simulink model "FuelSecondary_harness"  (Simulink 7.7)
settings: Solver=FixedStepDiscrete  SolverMode=SingleTasking  StartTime=0.0  StopTime=100  FixedStep=srate  RelTol=1e-3
InitFcn:
  | if signalbuilder('FuelSecondary_harness/Signal_Builder','activegroup') == 1
  |   CD_FUEL_SECONDARY_FUNCTION.DataType = 'uint8';
  |   CD_FUEL_SECONDARY_FUNCTION.Value = 255;
  |   CD_FUEL_SECONDARY_FEEDBACK_FUNCTION.DataType = 'uint8';
  |   CD_FUEL_SECONDARY_FEEDBACK_FUNCTION.Value = 255;
  | elseif signalbuilder('FuelSecondary_harness/Signal_Builder','activegroup') == 3
  |   CD_FUEL_SECONDARY_FUNCTION.DataType = 'uint8';
  |   CD_FUEL_SECONDARY_FUNCTION.Value = 255;
  |   CD_FUEL_SECONDARY_FEEDBACK_FUNCTION.DataType = 'uint8';
  |   CD_FUEL_SECONDARY_FEEDBACK_FUNCTION.Value = 255;
  | else
  |   CD_FUEL_SECONDARY_FUNCTION.DataType = 'uint8';
  |   CD_FUEL_SECONDARY_FUNCTION.Value = 0;
  |   CD_FUEL_SECONDARY_FEEDBACK_FUNCTION.DataType = 'uint8';
  |   CD_FUEL_SECONDARY_FEEDBACK_FUNCTION.Value = 0;
  | end
  | 
  | if signalbuilder('FuelSecondary_harness/Signal_Builder','activegroup') == 3
  |   CD_ECU_FUNCTION.DataType = 'uint8';
  |   CD_ECU_FUNCTION.Value = 0;
  | else
  |   CD_ECU_FUNCTION.DataType = 'uint8';
  |   CD_ECU_FUNCTION.Value = 255;
  | end
undefined symbols (not defined in the file): ACTIVE, CD_ECU_HOLD_DEBOUNCE_ERROR_ON, CD_FUEL_SECONDARY_AFBK_GAIN, ENGINE_CRANKING, ENGINE_OFF, FULL_ON, INACTIVE, NON_FUNCTIONAL, NORMAL, OORL, SHUTDOWN, sigbuilder_block, srate, SYS_NORMAL
libraries: simulink x3, MX_Library x1
Description:
  | Determines the state of the output and error coditions for the fuel secondary output.
CloseFcn:
  | rtwprivate ssgencode ModelCloseRequest sle_main_controller
settings Model: Creator=smindeman  LastModifiedBy=aliebel  ModifiedComment=smindema -- Wed Mar 08 09:39:08 2006 -- Version 1.339  RecordCoverage=on  CovPath=FuelSec_ECUHold/Solenoid  CovMetricSettings=dcmw  CovHTMLOptions=-aTS=1 -bRG=1 -bTC=1 -hTR=0 -nFC=0 -scm=1 -bcm=1 -xEv=0  covSaveCumulativeToWorkspaceVar=off  CovModelRefEnable=off
settings Model: ModifiedHistory=|
  | smindema -- Wed Mar 08 09:39:08 2006 -- Version 1.339
  | 
  | 
  | smindema -- Thu Mar 02 13:09:33 2006 -- Version 1.338
  | updated model per model review comments.
settings MATStruct: SampleTime=0.01  Offset=0  Priority=[1.0]
settings DataIOCC: LimitDataPoints=off  SaveOutput=off  SaveTime=off
settings OptimizationCC: BlockReduction=off  InlineParams=on  ExpressionFolding=off  StateBitsets=on  DataBitsets=on  UseTempVars=on  InitFltsAndDblsToZero=on  NoFixptDivByZeroProtection=on  EfficientFloat2IntCast=on  OptimizeModelRefInitCode=on
settings DebuggingCC: SaveWithParameterizedLinksMsg=none  MultiTaskDSMMsg=warning  MultiTaskCondExecSysMsg=none  IntegerOverflowMsg=none  ModelReferenceCSMismatchMessage=warning
settings HardwareCC: ProdBitPerInt=16  ProdBitPerPointer=16  ProdIntDivRoundTo=Zero  ProdEndianess=BigEndian  ProdWordSize=16  ProdHWDeviceType=Motorola HC12
settings ModelReferenceCC: ModelReferenceNumInstancesAllowed=Single
settings RTWCC: SystemTargetFile=ert.tlc  GenCodeOnly=on  TemplateMakefile=ert_default_tmf  Description=Real-Time Workshop Embedded Coder (no auto configuration)  GenerateReport=on  RetainRTWFile=on  ProcessScript=ert_make_rtw_hook  IncludeHyperlinkInReport=on  LaunchReport=on  IncludeERTFirstTime=on
settings RTWCC: CustomHeaderCode=|
  | #include "cpp_req_defines.h"
  | #include "hw_fin.h"
  | #include "cdata.h"
settings CodeAppCC: IgnoreCustomStorageClasses=off  DefineNamingRule=UpperCase
settings ERTTargetCC: TargetFcnLib=ansi_tfl_tmw.mat  FunctionExecutionProfile=off  MultiwordLength=2048  GenerateSampleERTMain=on  IncludeMdlTerminateFcn=off  SuppressErrorStatus=on  SupportAbsoluteTime=off  SupportNonFinite=off  SupportComplex=off  PurelyIntegerCode=on  ERTCustomFileTemplate=gen_rtw_req_defines_h.tlc  GlobalDataDefinition=InSeparateSourceFile  GlobalDataReference=InSeparateHeaderFile  ConvertIfToSwitch=off

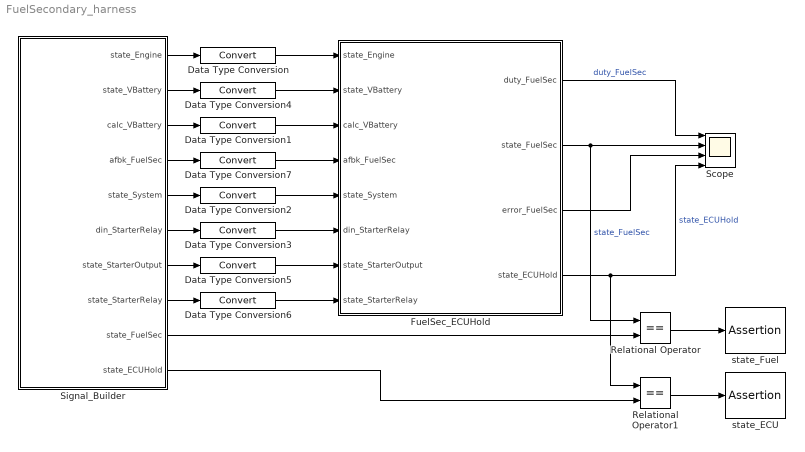
== system FuelSecondary_harness ==
  Data Type Conversion{,1..7} (8 alike) : DataTypeConversion
  FuelSec_ECUHold : Subsystem  TreatAsAtomicUnit=on  SystemSampleTime=srate  RTWFileName=mod_Outputs
      settings: RTWSystemCode=Function  RTWFileNameOpts=User specified
  Relational Operator : RelationalOperator  Operator===  OutDataTypeStr=boolean
  Relational Operator1 : RelationalOperator  Operator===  OutDataTypeStr=boolean
  Scope : Scope  NumInputPorts=4
      settings: TimeRange=100  YMin=0~0~-1~-5  YMax=1~8~1~5  MaxDataPoints=50000
  Signal_Builder : Subsystem  Tag=STV Subsys  LoadFcn=sigbuilder_block('load');  StartFcn=sigbuilder_block('start');  StopFcn=sigbuilder_block('stop');  ClipboardFcn=sigbuilder_block('clipboard');  mask(Sigbuilder block){}
      mask help: Sigbuilder GUI
      mask init:
      | if ~strcmp(get_param(bdroot(gcbh),'SimulationStatus'),'stopped') tuvar = sigbuilder_block('maskInit'); end
      settings: CopyFcn=sigbuilder_block('copy');  DeleteFcn=sigbuilder_block('delete');  ModelCloseFcn=sigbuilder_block('modelClose');  PreSaveFcn=sigbuilder_block('preSave');  NameChangeFcn=sigbuilder_block('namechange');  OpenFcn=sigbuilder_block('open',[579.75 151.5 804.75 557.25 ]);  CloseFcn=sigbuilder_block('close');
      mask Display: plot(0,0,100,100,[10,10,40,40,10],[80,20,20,80,80],[40,10],[50,50], [40,27,10],[65,72,56],[40,25,25,10],[28,28,43,43]);
  state_ECU : Assertion  Enabled=off
  state_Fuel : Assertion  Enabled=off
  wires:
  FuelSec_ECUHold/1(duty_FuelSec) -> Scope/1  "duty_FuelSec"
  FuelSec_ECUHold/2(state_FuelSec) -> Scope/2, Relational Operator/1  "state_FuelSec"
  Signal_Builder/1(state_Engine) -> Data Type Conversion/1
  Data Type Conversion/1 -> FuelSec_ECUHold/1(state_Engine)
  Signal_Builder/2(state_VBattery) -> Data Type Conversion4/1
  Data Type Conversion4/1 -> FuelSec_ECUHold/2(state_VBattery)
  Signal_Builder/3(calc_VBattery) -> Data Type Conversion1/1
  Data Type Conversion1/1 -> FuelSec_ECUHold/3(calc_VBattery)
  Data Type Conversion2/1 -> FuelSec_ECUHold/5(state_System)
  Data Type Conversion3/1 -> FuelSec_ECUHold/6(din_StarterRelay)
  Data Type Conversion5/1 -> FuelSec_ECUHold/7(state_StarterOutput)
  Data Type Conversion6/1 -> FuelSec_ECUHold/8(state_StarterRelay)
  FuelSec_ECUHold/4(state_ECUHold) -> Relational Operator1/1, Scope/4  "state_ECUHold"
  Relational Operator/1 -> state_Fuel/1
  Relational Operator1/1 -> state_ECU/1
  Signal_Builder/9(state_FuelSec) -> Relational Operator/2
  Signal_Builder/10(state_ECUHold) -> Relational Operator1/2
  Signal_Builder/8(state_StarterRelay) -> Data Type Conversion6/1
  Signal_Builder/7(state_StarterOutput) -> Data Type Conversion5/1
  Signal_Builder/6(din_StarterRelay) -> Data Type Conversion3/1
  Signal_Builder/5(state_System) -> Data Type Conversion2/1
  Signal_Builder/4(afbk_FuelSec) -> Data Type Conversion7/1
  Data Type Conversion7/1 -> FuelSec_ECUHold/4(afbk_FuelSec)
  FuelSec_ECUHold/3(error_FuelSec) -> Scope/3

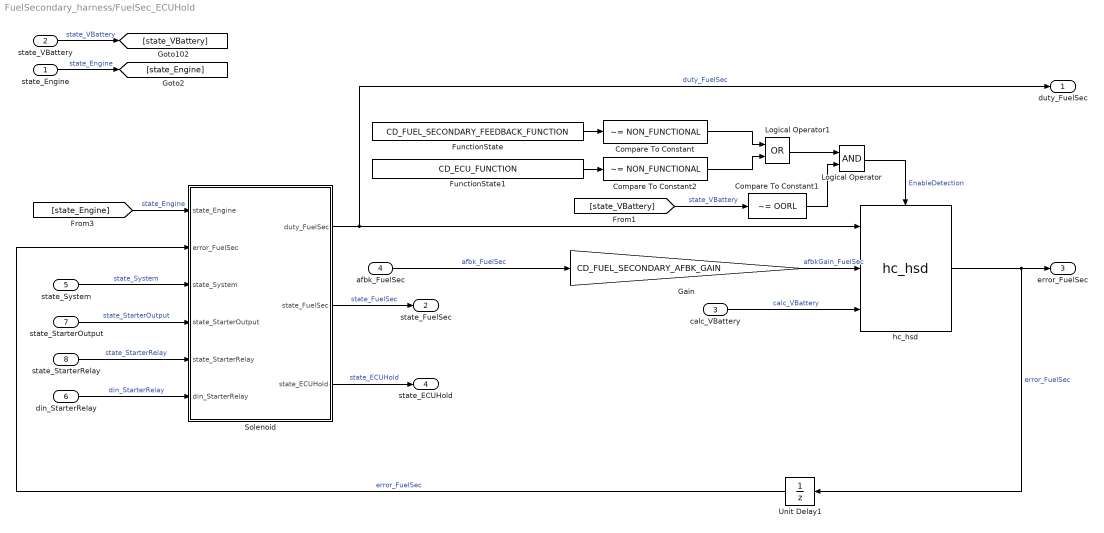
== system FuelSecondary_harness/FuelSec_ECUHold ==
  state_Engine : Inport  OutDataTypeStr=uint8
  state_VBattery : Inport  Port=2  OutDataTypeStr=uint8
  calc_VBattery : Inport  Port=3
  afbk_FuelSec : Inport  Port=4  OutDataTypeStr=uint16
  state_System : Inport  Port=5  OutDataTypeStr=uint8
  din_StarterRelay : Inport  Port=6  OutDataTypeStr=boolean
  state_StarterOutput : Inport  Port=7  OutDataTypeStr=uint8
  state_StarterRelay : Inport  Port=8  OutDataTypeStr=uint8
  Compare To Constant : simulink/Logic and Bit Operations/Compare To Constant  SystemSampleTime=-1  relop=~=  const=NON_FUNCTIONAL  LogicOutDataTypeMode=boolean  ZeroCross=off
  Compare To Constant1 : simulink/Logic and Bit Operations/Compare To Constant  SystemSampleTime=-1  relop=~=  const=OORL  LogicOutDataTypeMode=boolean  ZeroCross=off
  Compare To Constant2 : simulink/Logic and Bit Operations/Compare To Constant  SystemSampleTime=-1  relop=~=  const=NON_FUNCTIONAL  LogicOutDataTypeMode=boolean  ZeroCross=off
  FunctionState : Constant  Value=CD_FUEL_SECONDARY_FEEDBACK_FUNCTION  OutDataTypeStr=uint8
  FunctionState1 : Constant  Value=CD_ECU_FUNCTION  OutDataTypeStr=uint8
  Gain : Gain  Gain=CD_FUEL_SECONDARY_AFBK_GAIN  ParamDataTypeStr=fixdt(0,16,8)  OutDataTypeStr=fixdt(0,16,8)
  Logical Operator : Logic  AllPortsSameDT=off  OutDataTypeStr=boolean  SampleTime=srate
  Logical Operator1 : Logic  Operator=OR  AllPortsSameDT=off  OutDataTypeStr=boolean  SampleTime=srate
  Solenoid : Stateflow chart  TreatAsAtomicUnit=on
  Unit Delay1 : UnitDelay  SampleTime=srate
      settings: AttributesFormatString=<initial=%<X0>>\n<tsample=%<SampleTime>>
  hc_hsd : MX_Library/hc_hsd  SystemSampleTime=-1  STB_DB_CNT=CD_FUEL_SECONDARY_DEBOUNCE_SHORT_TO_BATTERY  STG_DB_CNT=CD_FUEL_SECONDARY_DEBOUNCE_SHORT_TO_GROUND  OPEN_DB_CNT=CD_FUEL_SECONDARY_DEBOUNCE_OPEN_CIRCUIT
  duty_FuelSec : Outport
  state_FuelSec : Outport  Port=2  OutDataTypeStr=uint8
  error_FuelSec : Outport  Port=3  OutDataTypeStr=uint8
  state_ECUHold : Outport  Port=4  OutDataTypeStr=uint8
  wires:
  Solenoid/2(state_FuelSec) -> state_FuelSec/1  "state_FuelSec"
  state_System/1 -> Solenoid/3(state_System)  "state_System"
  state_Engine/1 -> [state_Engine]  "state_Engine"
  state_VBattery/1 -> [state_VBattery]  "state_VBattery"
  Logical Operator/1 -> hc_hsd/Enable  "EnableDetection"
  Compare To Constant1/1 -> Logical Operator/2
  Logical Operator1/1 -> Logical Operator/1
  [state_VBattery] -> Compare To Constant1/1  "state_VBattery"
  Gain/1 -> hc_hsd/2  "afbkGain_FuelSec"
  Unit Delay1/1 -> Solenoid/2(error_FuelSec)  "error_FuelSec"
  Solenoid/1(duty_FuelSec) -> duty_FuelSec/1, hc_hsd/1  "duty_FuelSec"
  hc_hsd/1 -> error_FuelSec/1, Unit Delay1/1  "error_FuelSec"
  afbk_FuelSec/1 -> Gain/1  "afbk_FuelSec"
  calc_VBattery/1 -> hc_hsd/3  "calc_VBattery"
  [state_Engine] -> Solenoid/1(state_Engine)  "state_Engine"
  Solenoid/3(state_ECUHold) -> state_ECUHold/1  "state_ECUHold"
  FunctionState1/1 -> Compare To Constant2/1
  Compare To Constant2/1 -> Logical Operator1/2
  Compare To Constant/1 -> Logical Operator1/1
  FunctionState/1 -> Compare To Constant/1
  state_StarterOutput/1 -> Solenoid/4(state_StarterOutput)  "state_StarterOutput"
  state_StarterRelay/1 -> Solenoid/5(state_StarterRelay)  "state_StarterRelay"
  din_StarterRelay/1 -> Solenoid/6(din_StarterRelay)  "din_StarterRelay"

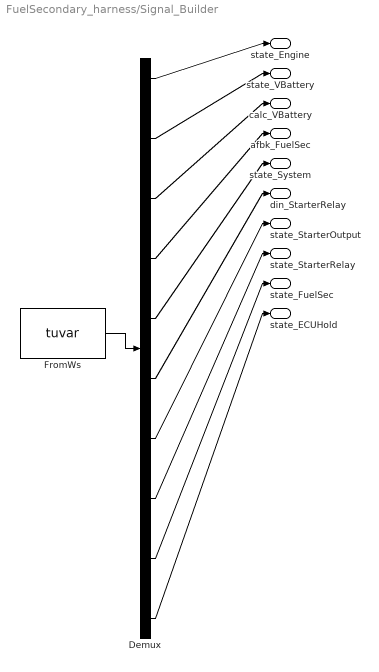
== system FuelSecondary_harness/Signal_Builder ==
  Demux : Demux  Tag=STV Demux  Outputs=10
  FromWs : FromWorkspace  Tag=STV FromWs  VariableName=tuvar  SampleTime=0  SigBuilderData=DataTag0  VnvData=DataTag1
      SigBuilderData=|
      | common.afterFinalStr = 'Extrapolate'
      | common.sampleTime = 0
      | dataSet(1).timeRange = [0 100]
      | dataSet(1).name = 'T1-NONFUNC'
      | dataSet(2).timeRange = [0 100]
      | dataSet(2).name = 'T2-NORMAL'
      | dataSet(3).timeRange = [0 100]
      | dataSet(3).name = 'T3-ECU'
      | sbobj.Groups(1).Name = 'T1-NONFUNC'
      | sbobj.Groups(1).Signals(1).Name = 'state_Engine'
      | sbobj.Groups(1).Signals(1).XData = [0 10.2 10.2 20 20 30 30 40 40 43.3 43.3 45.3 45.3 46.4 46.4 50 50 53.9 53.9 56.4 56.4 59.1 59.1 63.2 63.2 64.5 64.5 75.8 75.8 83.6 83.6 100]
      | sbobj.Groups(1).Signals(1).YData = [0 0 2 2 3 3 15 15 1 1 2 2 3 3 4 4 1 1 2 2 3 3 1 1 2 2 1 1 2 2 1 1]
      | sbobj.Groups(1).Signals(2).Name = 'state_VBattery'
      | sbobj.Groups(1).Signals(2).XData = [0 58.2 58.2 65.1 65.1 100]
      | sbobj.Groups(1).Signals(2).YData = [8 8 7 7 8 8]
      | sbobj.Groups(1).Signals(3).Name = 'calc_VBattery'
      | sbobj.Groups(1).Signals(3).XData = [0 72.6 72.6 80.6 80.6 100]
      | sbobj.Groups(1).Signals(3).YData = [0 0 1 1 0 0]
      | sbobj.Groups(1).Signals(4).Name = 'afbk_FuelSec'
      | sbobj.Groups(1).Signals(4).XData = [0 100]
      | sbobj.Groups(1).Signals(4).YData = [0 0]
      | sbobj.Groups(1).Signals(5).Name = 'state_System'
      | sbobj.Groups(1).Signals(5).XData = [0 3.6 3.6 5.7 5.7 60.7 60.7 62.1 62.1 100]
      | sbobj.Groups(1).Signals(5).YData = [1 1 0 0 1 1 0 0 1 1]
      | sbobj.Groups(1).Signals(6).Name = 'din_StarterRelay'
      | sbobj.Groups(1).Signals(6).XData = [0 100]
      | sbobj.Groups(1).Signals(6).YData = [0 0]
      | sbobj.Groups(1).Signals(7).Name = 'state_StarterOutput'
      | sbobj.Groups(1).Signals(7).XData = [0 100]
      | sbobj.Groups(1).Signals(7).YData = [8 8]
      | sbobj.Groups(1).Signals(8).Name = 'state_StarterRelay'
      | sbobj.Groups(1).Signals(8).XData = [0 100]
      | sbobj.Groups(1).Signals(8).YData = [8 8]
      | sbobj.Groups(1).Signals(9).Name = 'state_FuelSec'
      | sbobj.Groups(1).Signals(9).XData = [0 100]
      | sbobj.Groups(1).Signals(9).YData = [0 0]
      | sbobj.Groups(1).Signals(10).Name = 'state_ECUHold'
      | sbobj.Groups(1).Signals(10).XData = [0 100]
      | sbobj.Groups(1).Signals(10).YData = [0 0]
      | sbobj.Groups(2).Name = 'T2-NORMAL'
      | sbobj.Groups(2).Signals(1).Name = 'state_Engine'
      | sbobj.Groups(2).Signals(1).XData = [0 10.2 10.2 20 20 30 30 40 40 43.3 43.3 45.3 45.3 46.4 46.4 50 50 53.9 53.9 56.4 56.4 59.1 59.1 63.2 63.2 64.5 64.5 75.8 75.8 83.6 83.6 100]
      | sbobj.Groups(2).Signals(1).YData = [0 0 2 2 3 3 15 15 1 1 2 2 3 3 4 4 1 1 2 2 3 3 1 1 2 2 1 1 2 2 1 1]
      | sbobj.Groups(2).Signals(2).Name = 'state_VBattery'
      | sbobj.Groups(2).Signals(2).XData = [0 77.4 77.4 83.2 83.2 100]
      | sbobj.Groups(2).Signals(2).YData = [8 8 22 22 8 8]
      | sbobj.Groups(2).Signals(3).Name = 'calc_VBattery'
      | sbobj.Groups(2).Signals(3).XData = [0 76.6 76.6 83.2 83.2 100]
      | sbobj.Groups(2).Signals(3).YData = [14.5 14.5 5 5 14.5 14.5]
      | sbobj.Groups(2).Signals(4).Name = 'afbk_FuelSec'
      | sbobj.Groups(2).Signals(4).XData = [0 10.21 10.21 30.01 30.01 43.3 43.3 46.41 46.41 51 51 65.8 65.8 83.2 83.2 100]
      | sbobj.Groups(2).Signals(4).YData = [0 0 663 663 0 0 663 663 0 0 336 336 0 0 663 663]
      | sbobj.Groups(2).Signals(5).Name = 'state_System'
      | sbobj.Groups(2).Signals(5).XData = [0 3.6 3.6 5.7 5.7 60.7 60.7 62.1 62.1 94 94 96.2 96.2 100]
      | sbobj.Groups(2).Signals(5).YData = [1 1 0 0 1 1 0 0 1 1 0 0 1 1]
      | sbobj.Groups(2).Signals(6).Name = 'din_StarterRelay'
      | sbobj.Groups(2).Signals(6).XData = [0 100]
      | sbobj.Groups(2).Signals(6).YData = [0 0]
      | sbobj.Groups(2).Signals(7).Name = 'state_StarterOutput'
      | sbobj.Groups(2).Signals(7).XData = [0 100]
      | sbobj.Groups(2).Signals(7).YData = [8 8]
      | sbobj.Groups(2).Signals(8).Name = 'state_StarterRelay'
      | sbobj.Groups(2).Signals(8).XData = [0 100]
      | sbobj.Groups(2).Signals(8).YData = [8 8]
      | sbobj.Groups(2).Signals(9).Name = 'state_FuelSec'
      | sbobj.Groups(2).Signals(9).XData = [0 10.2 10.2 30 30 43.3 43.3 46.41 46.41 51.22 51.22 60.7 60.7 62.11 62.11 77.41 77.41 77.42 77.42 94 94 96.21 96.21 100]
      | sbobj.Groups(2).Signals(9).YData = [0 0 1 1 0 0 1 1 0 0 7 7 0 0 7 7 0 0 1 1 0 0 5 5]
      | sbobj.Groups(2).Signals(10).Name = 'state_ECUHold'
      | sbobj.Groups(2).Signals(10).XData = [0 100]
      | sbobj.Groups(2).Signals(10).YData = [0 0]
      | sbobj.Groups(3).Name = 'T3-ECU'
      | sbobj.Groups(3).Signals(1).Name = 'state_Engine'
      | sbobj.Groups(3).Signals(1).XData = [0 3.8 3.8 7.3 7.3 49.1 49.1 54.1 54.1 60.7 60.7 65.6 65.6 100]
      | sbobj.Groups(3).Signals(1).YData = [1 1 2 2 1 1 4 4 1 1 15 15 1 1]
      | sbobj.Groups(3).Signals(2).Name = 'state_VBattery'
      | sbobj.Groups(3).Signals(2).XData = [0 71.6 71.6 75.6 75.6 100]
      | sbobj.Groups(3).Signals(2).YData = [8 8 22 22 8 8]
      | sbobj.Groups(3).Signals(3).Name = 'calc_VBattery'
      | sbobj.Groups(3).Signals(3).XData = [0 71.8 71.8 75.6 75.6 100]
      | sbobj.Groups(3).Signals(3).YData = [14 14 6 6 14 14]
      | sbobj.Groups(3).Signals(4).Name = 'afbk_FuelSec'
      | sbobj.Groups(3).Signals(4).XData = [0 3.8 3.8 12.7 12.7 24.3 24.3 29.8 29.8 35.4 35.4 39 39 43.7 43.7 49.1 49.1 50 50 75.8 75.8 100]
      | sbobj.Groups(3).Signals(4).YData = [0 0 663 663 0 0 663 663 0 0 663 663 0 0 663 663 0 0 336 336 663 663]
      | sbobj.Groups(3).Signals(5).Name = 'state_System'
      | sbobj.Groups(3).Signals(5).XData = [0 3.6 12.7 12.7 15.1 15.1 100]
      | sbobj.Groups(3).Signals(5).YData = [1 1 1 0 0 1 1]
      | sbobj.Groups(3).Signals(6).Name = 'din_StarterRelay'
      | sbobj.Groups(3).Signals(6).XData = [0 10 10 100]
      | sbobj.Groups(3).Signals(6).YData = [1 1 0 0]
      | sbobj.Groups(3).Signals(7).Name = 'state_StarterOutput'
      | sbobj.Groups(3).Signals(7).XData = [0 15.1 15.1 20.7 20.7 29.8 29.8 35.4 35.4 100]
      | sbobj.Groups(3).Signals(7).YData = [8 8 7 7 8 8 7 7 8 8]
      | sbobj.Groups(3).Signals(8).Name = 'state_StarterRelay'
      | sbobj.Groups(3).Signals(8).XData = [0 19.4 19.4 24.3 24.3 39 39 43.7 43.7 100]
      | sbobj.Groups(3).Signals(8).YData = [8 8 7 7 8 8 7 7 8 8]
      | sbobj.Groups(3).Signals(9).Name = 'state_FuelSec'
      | sbobj.Groups(3).Signals(9).XData = [0 100]
      | sbobj.Groups(3).Signals(9).YData = [0 0]
      | sbobj.Groups(3).Signals(10).Name = 'state_ECUHold'
      | sbobj.Groups(3).Signals(10).XData = [0 3.8 3.8 12.7 12.7 24.3 24.3 29.8 29.8 35.4 35.4 39 39 43.7 43.7 49.1 49.1 50.22 50.22 60.7 60.7 65.62 65.62 71.61 71.61 71.82 71.82 80.6 100]
      | sbobj.Groups(3).Signals(10).YData = [0 0 1 1 0 0 1 1 0 0 1 1 0 0 1 1 0 0 7 7 0 0 7 7 0 0 1 1 1]
  state_Engine : Outport  Tag=STV Outport
  state_VBattery : Outport  Tag=STV Outport  Port=2
  calc_VBattery : Outport  Tag=STV Outport  Port=3
  afbk_FuelSec : Outport  Tag=STV Outport  Port=4
  state_System : Outport  Tag=STV Outport  Port=5
  din_StarterRelay : Outport  Tag=STV Outport  Port=6
  state_StarterOutput : Outport  Tag=STV Outport  Port=7
  state_StarterRelay : Outport  Tag=STV Outport  Port=8
  state_FuelSec : Outport  Tag=STV Outport  Port=9
  state_ECUHold : Outport  Tag=STV Outport  Port=10
  wires:
  FromWs/1 -> Demux/1
  Demux/1 -> state_Engine/1
  Demux/2 -> state_VBattery/1
  Demux/3 -> calc_VBattery/1
  Demux/4 -> afbk_FuelSec/1
  Demux/5 -> state_System/1
  Demux/6 -> din_StarterRelay/1
  Demux/7 -> state_StarterOutput/1
  Demux/8 -> state_StarterRelay/1
  Demux/9 -> state_FuelSec/1
  Demux/10 -> state_ECUHold/1

== stateflow chart FuelSec_ECUHold/Solenoid ==
  state NON_FUNCTIONAL
    en:duty_FuelSec = INACTIVE;
    en:state_FuelSec = INACTIVE;
    en:state_ECUHold = INACTIVE;
  state FUEL_HOLD
    state ACTIVE
      state ACTIVE
        en:duty_FuelSec = FULL_ON;
        en:state_FuelSec = ACTIVE;
      state INACTIVE
        en:duty_FuelSec = INACTIVE;
        en:state_FuelSec = INACTIVE;
      (default) -> INACTIVE
      INACTIVE -> FUEL_HOLD.ACTIVE.ACTIVE : [state_Engine == ENGINE_CRANKING]
      FUEL_HOLD.ACTIVE.ACTIVE -> INACTIVE : [(state_Engine == SHUTDOWN)...
          | || (state_Engine == ENGINE_OFF)]
    state ERROR
      en:duty_FuelSec = INACTIVE;
      en:state_FuelSec = error_FuelSec;
    FUEL_HOLD.ACTIVE -> FUEL_HOLD.ERROR : [(error_FuelSec != NORMAL)]
    FUEL_HOLD.ERROR -> FUEL_HOLD.ACTIVE : [(error_FuelSec == NORMAL)]
    (default) -> FUEL_HOLD.ACTIVE
  state ECU_HOLD
    state NORMAL
      state ACTIVE
        en:duty_FuelSec = FULL_ON;
        en:state_ECUHold = ACTIVE;
      state CHECK_ERROR_ON
        en:duty_FuelSec = INACTIVE;
        en:state_ECUHold = INACTIVE;
        en:debounceCount = 0;
        du:debounceCount++;
      note: Only go active if the starter output is inactive unless
          | we are in a cranking state.  We do not want the machine
          | to start cranking once key is on if the starter is shorted.
      CHECK_ERROR_ON -> ECU_HOLD.NORMAL.ACTIVE : [(debounceCount >= CD_ECU_HOLD_DEBOUNCE_ERROR_ON)...
          | && (state_StarterOutput == NORMAL)...
          | && (state_StarterRelay == NORMAL)...
          | && ((din_StarterRelay == INACTIVE) || (state_Engine == ENGINE_CRANKING))...
          | && (state_Engine != ENGINE_OFF)]
      (default) -> CHECK_ERROR_ON
      ECU_HOLD.NORMAL.ACTIVE -> CHECK_ERROR_ON : [(state_StarterOutput != NORMAL)...
          | || (state_StarterRelay != NORMAL)...
          | || (state_Engine == ENGINE_OFF)]
    state ERROR
      en:duty_FuelSec = INACTIVE;
      en:state_ECUHold = error_FuelSec;
    NORMAL -> ECU_HOLD.ERROR : [(error_FuelSec != NORMAL)]
    ECU_HOLD.ERROR -> NORMAL : [(error_FuelSec == NORMAL)]
    (default) -> NORMAL
  NON_FUNCTIONAL -> FUEL_HOLD [order 2] : [(CD_FUEL_SECONDARY_FUNCTION != NON_FUNCTIONAL)...
      | && (state_System == SYS_NORMAL)]
  FUEL_HOLD -> NON_FUNCTIONAL : [(state_System != SYS_NORMAL)]
  (default) -> NON_FUNCTIONAL
  ECU_HOLD -> NON_FUNCTIONAL : [(state_System != SYS_NORMAL)...
      | || (state_Engine == SHUTDOWN)]
  NON_FUNCTIONAL -> ECU_HOLD [order 1] : [(CD_ECU_FUNCTION != NON_FUNCTIONAL)...
      | && (state_System == SYS_NORMAL)...
      | && (state_Engine != SHUTDOWN)]
  data: state_Engine input uint8; error_FuelSec input uint8; duty_FuelSec output fixdt(0,16,16); CD_FUEL_SECONDARY_FUNCTION parameter uint8; FULL_ON parameter fixdt(0,16,16); NORMAL parameter uint8 =8; INACTIVE parameter uint8 =8; SHUTDOWN parameter uint8 =8; ENGINE_CRANKING parameter uint8; SYS_NORMAL parameter uint8; state_System input uint8; ENGINE_OFF parameter uint8; state_FuelSec output uint8; ACTIVE parameter uint8; NON_FUNCTIONAL parameter uint8; CD_ECU_FUNCTION parameter uint8; CD_ECU_HOLD_DEBOUNCE_ERROR_ON parameter uint16; state_ECUHold output uint8; debounceCount local uint16; state_StarterOutput input uint8; state_StarterRelay input uint8; din_StarterRelay input boolean
